simulink model "ex4_s"  (Simulink 7.9)
settings: Solver=ode45  StartTime=0.0  StopTime=10.0  RelTol=1e-3
settings Model: Creator=Theodor  LastModifiedBy=Theodor
settings DebuggingCC: SolverPrmCheckMsg=none

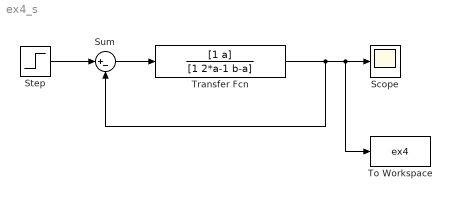
== system ex4_s ==
  Scope : Scope
  Step : Step  SampleTime=0
  Sum : Sum  Inputs=|+-
  To Workspace : ToWorkspace  VariableName=ex4  SampleTime=-1
  Transfer Fcn : TransferFcn  Numerator=[1 a]  Denominator=[1 2*a-1 b-a]  mask{a=4, b=36}
      mask CallbackString:
      | if str2num(get_param(gcb,'a')) < 0
      |     error('parametru negativ');
      | end|if str2num(get_param(gcb,'b')) < 0
      |     error('parametru negativ');
      | end
  wires:
  Transfer Fcn/1 -> Sum/2, Scope/1, To Workspace/1
  Step/1 -> Sum/1
  Sum/1 -> Transfer Fcn/1
